simulink library "Open_Surface"  (Simulink 8.2)
settings: Solver=ode45  StartTime=0.0  StopTime=10.0  RelTol=1e-3
libraries: carnot x2
settings Model: Creator=lena.frank  LastModifiedBy=drhf

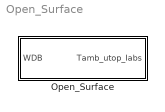
== system Open_Surface ==
  Open_Surface : Subsystem  mask(open surface){albedo=0.6}
      mask prompts: albedo "albedo of the surface [0..1]"
      mask help: This is a surface-model for ground storages. It describes the absorption of solar radiation and the heat losses by wind.
      mask init:
      | albedo = min(1, max(0, albedo));
      mask Help: web(fullfile(path_carnot('help'),'Open_Surface.html'),'-helpbrowser')

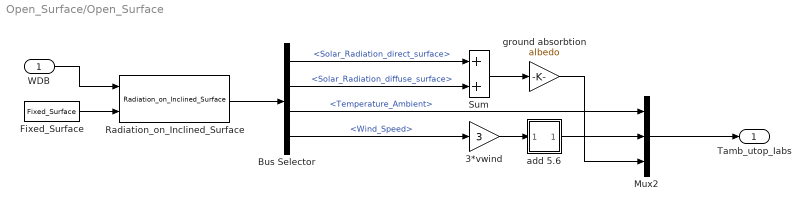
== system Open_Surface/Open_Surface ==
  WDB : Inport
  3*vwind : Gain  Gain=3  SaturateOnIntegerOverflow=on  OutDataTypeStr=Inherit: Same as input  ParamDataTypeStr=Inherit: Same as input
  Bus Selector : BusSelector  OutputSignals=Solar_Radiation_direct_surface,Solar_Radiation_diffuse_surface,Temperature_Ambient,Wind_Speed
  Fixed_Surface : carnot/Weather/Fixed_Surface  colangle=0  colazi=0  colrot=0
  Mux2 : Mux  Inputs=3
  Radiation_on_Inclined_Surface : carnot/Weather/Radiation_on_Inclined_Surface  sky=Perez 1990  reflect=0.2
  Sum : Sum  Inputs=2  SaturateOnIntegerOverflow=on  InputSameDT=on  OutDataTypeStr=Inherit: Same as first input
  add 5.6 : Subsystem  mask(add constant){c=5.6}
      mask prompts: c "constant c"
      mask help: This block adds a constant c to each element of the input vector.
      mask Help: file:///constant.htm
      mask Display: disp('+c');
  ground absorbtion : Gain  Gain=albedo  SaturateOnIntegerOverflow=on  OutDataTypeStr=Inherit: Same as input  ParamDataTypeStr=Inherit: Same as input
  Tamb_utop_Iabs : Outport
  wires:
  Bus Selector/4 -> 3*vwind/1  "<Wind_Speed>"
  Mux2/1 -> Tamb_utop_Iabs/1
  add 5.6/1(Out1) -> Mux2/2
  3*vwind/1 -> add 5.6/1(In1)
  Sum/1 -> ground absorbtion/1
  Bus Selector/1 -> Sum/1  "<Solar_Radiation_direct_surface>"
  ground absorbtion/1 -> Mux2/3
  Bus Selector/3 -> Mux2/1  "<Temperature_Ambient>"
  Radiation_on_Inclined_Surface/1 -> Bus Selector/1
  Fixed_Surface/1 -> Radiation_on_Inclined_Surface/2
  WDB/1 -> Radiation_on_Inclined_Surface/1
  Bus Selector/2 -> Sum/2  "<Solar_Radiation_diffuse_surface>"

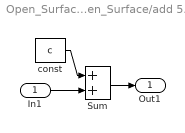
== system Open_Surface/Open_Surface/add 5.6 ==
  In1 : Inport
  Sum : Sum  SaturateOnIntegerOverflow=on  InputSameDT=on  OutDataTypeStr=Inherit: Same as first input
  const : Constant  Value=c
  Out1 : Outport
  wires:
  Sum/1 -> Out1/1
  In1/1 -> Sum/2
  const/1 -> Sum/1
